simulink model "Boat_model_next"  (Simulink 6.6)
settings: Solver=ode3  StartTime=0.0  StopTime=1000.0  FixedStep=1  RelTol=1e-3
libraries: simulink x2
settings Model: Creator=Administrator  LastModifiedBy=Administrator

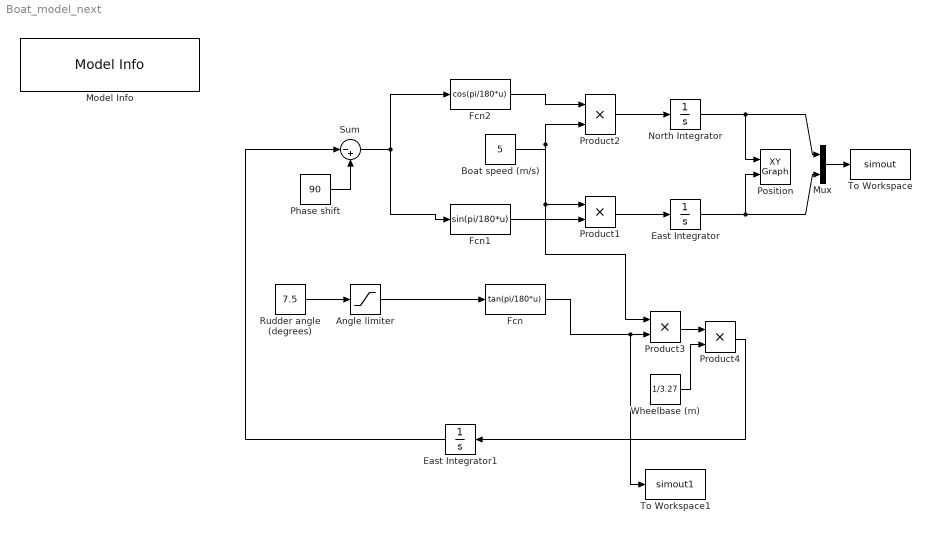
== system Boat_model_next ==
  Angle limiter : Saturate  UpperLimit=60  LowerLimit=-60
  Boat speed (m/s) : Constant  Value=5
  East Integrator : Integrator
  East Integrator1 : Integrator  Orientation=left
  Fcn : Fcn  Expr=tan(pi/180*u)
  Fcn1 : Fcn  Expr=sin(pi/180*u)
  Fcn2 : Fcn  Expr=cos(pi/180*u)
  Model Info : simulink/Model-Wide Utilities/Model Info  SystemSampleTime=-1  InitialBlockCM=None  BlockCM=None  Frame=on  DisplayStringWithTags=|  HorizontalTextAlignment=Center  LeftAlignmentValue=0.5  SourceBlockDiagram=Boat_model_next  TagMaxNumber=20
      | Kinematic model of the autoboat.
      | Version %<ModelVersion>
  Mux : Mux  Inputs=2
  North Integrator : Integrator
  Phase shift : Constant  Value=90
  Position : simulink/Sinks/XY Graph  SystemSampleTime=-1  xmin=-10000  xmax=10000  ymin=-10000  ymax=10000  st=-1
  Product{1..4} (4 alike) : Product  RndMeth=Zero
  Rudder angle (degrees) : Constant  Value=7.5
  Sum : Sum  Inputs=|-+
  To Workspace : ToWorkspace  VariableName=simout  SampleTime=-1  SaveFormat=Structure
  To Workspace1 : ToWorkspace  VariableName=simout1  SampleTime=-1  SaveFormat=Structure
  Wheelbase (m) : Constant  Value=1/3.27
  wires:
  Rudder angle (degrees)/1 -> Angle limiter/1
  North Integrator/1 -> Position/1, Mux/1
  Fcn2/1 -> Product2/1
  East Integrator/1 -> Position/2, Mux/2
  Fcn1/1 -> Product1/2
  Mux/1 -> To Workspace/1
  Product2/1 -> North Integrator/1
  Boat speed (m/s)/1 -> Product2/2, Product1/1, Product3/1
  Fcn/1 -> Product3/2, To Workspace1/1
  Wheelbase (m)/1 -> Product4/2
  Product3/1 -> Product4/1
  Sum/1 -> Fcn2/1, Fcn1/1
  Phase shift/1 -> Sum/2
  Product1/1 -> East Integrator/1
  Angle limiter/1 -> Fcn/1
  Product4/1 -> East Integrator1/1
  East Integrator1/1 -> Sum/1
